simulink model "fullBridgeConverter"  (R2019a)
settings: Solver=VariableStepAuto  StartTime=0.0  StopTime=0.1  RelTol=1e-3
libraries: powerlib x18, dspstat3 x1
settings Model: Creator=Toshıba  LastModifiedBy=Toshıba

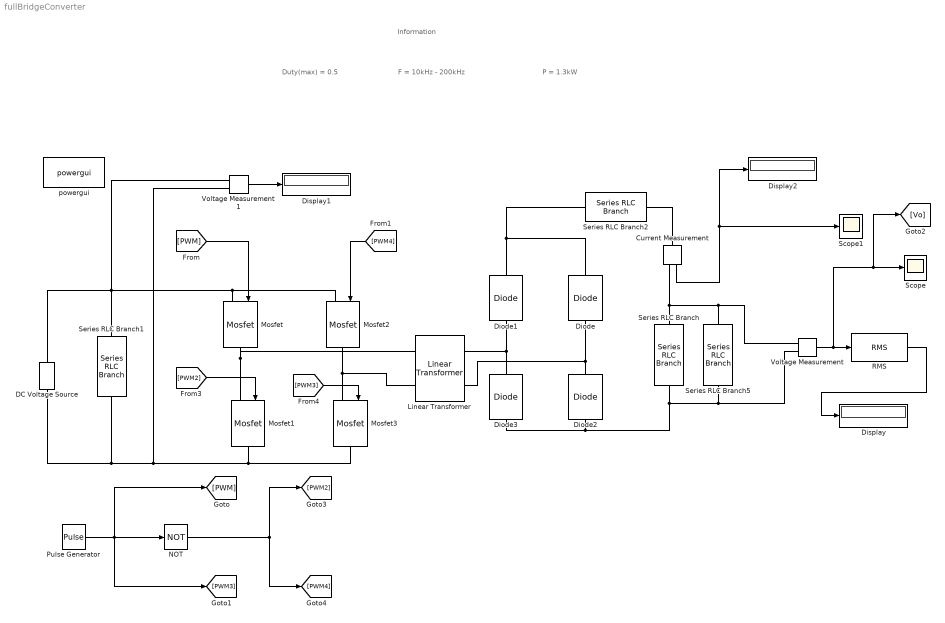
== system fullBridgeConverter ==
  note: P = 1.3kW
  note: F = 10kHz - 200kHz
  note: Information
  note: Duty(max) = 0.5
  Current Measurement : powerlib/Measurements/Current Measurement  PhasorSimulation=off  OutputType=Complex  PSBequivalent=0
      settings: SourceProductName=Simscape Electrical
  DC Voltage Source : powerlib/Electrical Sources/DC Voltage Source  Amplitude=220  Measurements=None
      settings: SourceProductName=Simscape Electrical
  Diode{,1..3} (4 alike) : powerlib/Power Electronics/Diode  Ron=0.001  Lon=0  Vf=0.5  IC=0  UseSnubber=0  Rs=500  Cs=250e-9  Measurements=off
      settings: SourceProductName=Simscape Electrical
  Display : Display
  Display1 : Display
  Display2 : Display
  Linear Transformer : powerlib/Elements/Linear Transformer  UNITS=SI  NominalPower=[ 13e2 200e3 ]  winding1=[220 0 0]  winding2=[72 0 0]  ThreeWindings=off  winding3=[3.15e+05 0.7938 0.084225]  RmLm=[1.0805e+06 2866]  Measurements=None  DataType=on
      settings: SourceProductName=Simscape Electrical
  Mosfet{,1..3} (4 alike) : powerlib/Power Electronics/Mosfet  Ron=0.1  Lon=0  Rd=0.01  Vfd=0  IC=0  Rs=1e5  Cs=inf  Measurements=off
      settings: SourceProductName=Simscape Electrical
  NOT : Logic  Operator=NOT  IconShape=distinctive  AllPortsSameDT=off  OutDataTypeStr=boolean
  Pulse Generator : DiscretePulseGenerator  PulseType=Time based  Period=5e-6  PulseWidth=50
  RMS : dspstat3/RMS  run=off  directionMode=Each column  dimension=1  InputProcessing=Columns as channels (frame based)  reset_popup=None
  Scope : Scope
  Scope1 : Scope
  Series RLC Branch : powerlib/Elements/Series RLC Branch  LConnTagsString=__new0  RConnTagsString=__new0  BranchType=C  Resistance=1  Inductance=1e-3  SetiL0=off  InitialCurrent=0  Capacitance=18.94e-6  Setx0=off  InitialVoltage=0  Measurements=None
      settings: SourceProductName=Simscape Electrical
  Series RLC Branch1 : powerlib/Elements/Series RLC Branch  LConnTagsString=__new0  RConnTagsString=__new0  BranchType=RC  Resistance=0.001  Inductance=1e-3  SetiL0=off  InitialCurrent=0  Capacitance=10e-6  Setx0=off  InitialVoltage=0  Measurements=None
      settings: SourceProductName=Simscape Electrical
  Series RLC Branch2 : powerlib/Elements/Series RLC Branch  LConnTagsString=__new0  RConnTagsString=__new0  BranchType=L  Resistance=1  Inductance=3.3e-6  SetiL0=off  InitialCurrent=0  Capacitance=1e-6  Setx0=off  InitialVoltage=0  Measurements=None
      settings: SourceProductName=Simscape Electrical
  Series RLC Branch5 : powerlib/Elements/Series RLC Branch  LConnTagsString=__new0  RConnTagsString=__new0  BranchType=R  Resistance=4  Inductance=1e-3  SetiL0=off  InitialCurrent=0  Capacitance=1e-6  Setx0=off  InitialVoltage=0  Measurements=None
      settings: SourceProductName=Simscape Electrical
  Voltage Measurement : powerlib/Measurements/Voltage Measurement  PhasorSimulation=off  OutputType=Complex  PSBequivalent=0
      settings: SourceProductName=Simscape Electrical
  Voltage Measurement1 : powerlib/Measurements/Voltage Measurement  PhasorSimulation=off  OutputType=Complex  PSBequivalent=0
      settings: SourceProductName=Simscape Electrical
  powergui : powerlib/powergui  Priority=1  SimulationMode=Continuous  SampleTime=1e-6  frequency=60  Iterations=50  frequencyindice=0  Pbase=100e6  ErrMax=1e-4  UnitsV=kV  UnitsW=MW  buscounter=0  FunctionMessages=off  echomessages=off  EnableUseOfTLC=off  CurrentSourceSwitches=off  DisableSnubberDevices=off  DisableRonSwitches=off  DisableVfSwitches=off  DisplayEquations=off  AutomaticDiscreteSolvers=off  SolverType=Tustin/Backward Euler (TBE)  Interpol=off  ExternalGateDelay=off  methode=off  Ts=100  x0status=blocks  SPID=on  SwTol=0  HookPort=off  NonlinearTolerance=0  nMaxIteration=15  ContinueOnMaxIteration=off  RestoreLinks=warning  ResistiveCurrentMeasurement=off  Frange=[0:2:500]  Ylog=off  Xlog=on  ShowGrid=off  save=off  variable=ZData  structure=0  ZoomFFT=off  StartTime=0.0  cycles=1  DisplayStyle=1  fundamental=60  FreqAxis=off  MaxFrequency=1000  frequencyindicesteady=1  RmsSteady=1  display=off
      settings: SourceProductName=Simscape Electrical
  wires:
  Voltage Measurement1/1 -> Display1/1
  Voltage Measurement/1 -> [Vo], Scope/1, RMS/1
  RMS/1 -> Display/1
  Current Measurement/1 -> Scope1/1, Display2/1
  [PWM3] -> Mosfet3/1
  [PWM4] -> Mosfet2/1
  [PWM] -> Mosfet/1
  [PWM2] -> Mosfet1/1
  Pulse Generator/1 -> [PWM3], [PWM], NOT/1
  NOT/1 -> [PWM4], [PWM2]
  connections:
  DC Voltage Source/LConn1 -- Voltage Measurement1/LConn2 -- Mosfet1/RConn1 -- Mosfet3/RConn1 -- Series RLC Branch1/RConn1
  DC Voltage Source/RConn1 -- Voltage Measurement1/LConn1 -- Series RLC Branch1/LConn1 -- Mosfet2/LConn1 -- Mosfet/LConn1
  Diode1/RConn1 -- Diode/RConn1 -- Series RLC Branch2/LConn1
  Series RLC Branch5/LConn1 -- Series RLC Branch/LConn1 -- Current Measurement/RConn1 -- Voltage Measurement/LConn1
  Mosfet/RConn1 -- Linear Transformer/LConn1 -- Mosfet1/LConn1
  Mosfet2/RConn1 -- Linear Transformer/LConn2 -- Mosfet3/LConn1
  Diode3/LConn1 -- Voltage Measurement/LConn2 -- Series RLC Branch5/RConn1 -- Series RLC Branch/RConn1 -- Diode2/LConn1
  Series RLC Branch2/RConn1 -- Current Measurement/LConn1
  Diode3/RConn1 -- Linear Transformer/RConn1 -- Diode1/LConn1
  Diode/LConn1 -- Linear Transformer/RConn2 -- Diode2/RConn1
